simulink model "package"  (R2018b)
settings: Solver=FixedStepDiscrete  StartTime=0.0  StopTime=10  FixedStep=Ts  RelTol=1e-3
PreLoadFcn:
  | Ts = 0.001;
InitFcn:
  | Ts = 0.001;
  | %mex controller.c;
undefined symbols (not defined in the file or in its folder): DiscIntNeverNeededParam, x2m
libraries: powerlib_meascontrol x6, motion x5, simulink x2, peGeneralControl x2
(part 2 of 2)

== matlab function package/profiles/hashem profile/TD/MATLAB Function ==
  data: x1 input; f output; x2 input; r input; h input
function f = fhan(x1, x2, r, h)

    d = r * h^2;
    a0 = h * x2;
    y = x1 + a0;
    a1 = sqrt(d * (d + 8 * abs(y)));
    a2 = a0 + sign(y) * (a1 - d) / 2;
    sy = (sign(y + d) - sign(y - d)) / 2;
    a = (a0 + y - a2) * sy + a2;
    sa = (sign(a + d) - sign(a - d)) / 2;
    f = -r * (a / d - sign(a)) * sa - r * sign(a);

end

== matlab function package/Subsystem/MATLAB Function ==
  data: x1 input; x1cal output; x2 input; x3 input; x2cal output
function [x1cal,x2cal] = fcnp(x1,x2,x3)

x3mn = 0.5;
x4s = 3;

x2cal = (1/24)*x3mn^3/x4s^2+x2^2/(2*x3mn) + x1;

x2max = x2+x3^2/(x4s*2);
x3max = x3mn;
x1cal = x3/x4s*(x2+(x3^2)/(3*x4s))+x2max*(x3max/x4s+x2max/x3max)/2 + x1;


% syms x1 x2 x4s x3mn
% x3 = x3mn;
% 
% x1cal = (1/24)*x3mn^3/x4s^2+x2^2/(2*x3mn) + x1;
% simplifyFraction(x1cal)
% 
% x2max = x2+x3^2/(x4s*2);
% x3max = x3mn;%sqrt((x2max)*x4s); min(x3mn,sqrt(abs(x2max)*x4s));
% x1cal = x3/x4s*(x2+(x3^2)/(3*x4s))+x2max*(x3max/x4s+x2max/x3max)/2 + x1;
% simplifyFraction(x1cal)
